simulink model "bio_matfunc_srp_torque_var"  (R2017b)
settings: Solver=VariableStepAuto  StartTime=0.0  StopTime=10.0  RelTol=1e-3
settings Model: Creator=ktrinh  LastModifiedBy=ktrinh

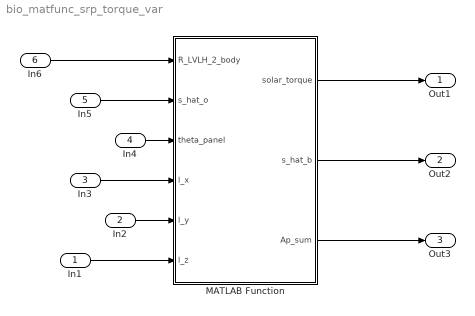
== system bio_matfunc_srp_torque_var ==
  In1 : Inport  OutDataTypeStr=double  PortDimensions=1
  In2 : Inport  Port=2  OutDataTypeStr=double  PortDimensions=1
  In3 : Inport  Port=3  OutDataTypeStr=double  PortDimensions=1
  In4 : Inport  Port=4  OutDataTypeStr=double  PortDimensions=1
  In5 : Inport  Port=5  OutDataTypeStr=double  PortDimensions=3
  In6 : Inport  Port=6  OutDataTypeStr=double  PortDimensions=[3,3]
  MATLAB Function : MATLAB Function  TreatAsAtomicUnit=on
  Out1 : Outport
  Out2 : Outport  Port=2
  Out3 : Outport  Port=3
  wires:
  In1/1 -> MATLAB Function/6(l_z)
  In2/1 -> MATLAB Function/5(l_y)
  In3/1 -> MATLAB Function/4(l_x)
  In4/1 -> MATLAB Function/3(theta_panel)
  In5/1 -> MATLAB Function/2(s_hat_o)
  MATLAB Function/1(solar_torque) -> Out1/1
  MATLAB Function/2(s_hat_b) -> Out2/1
  MATLAB Function/3(Ap_sum) -> Out3/1
  In6/1 -> MATLAB Function/1(R_LVLH_2_body)

== matlab function bio_matfunc_srp_torque_var/MATLAB Function ==
  data: R_LVLH_2_body input; solar_torque output; s_hat_o input; theta_panel input; l_x input; l_y input; l_z input; s_hat_b output; Ap_sum output
% function [solar_torque,s_hat_b] = srp_torque_var(R_LVLH_2_body,s_hat_o,theta_panel,l_x,l_y,l_z)
% %#codegen
% 
% Rob = R_LVLH_2_body;
% % this function calculates solar torque for a variable panel configuration
% % where the solar panels can rotate about the spacecraft y-axis
% % theta_panel is the angle in degrees that the panels are rotated from the
% % z axis -- i.e. theta_panel = 0 when panels are aligned normal to z axis
% 
% % Define constants
% SC = 1367;       % W/m^2, solar constant
% c = 3e8;         % m/s, speed of light
% q = 1;           % Reflectance
% 
% % Calculate an intermediate constant
% Fc = (SC/c)*(1+q);
% 
% % Define the surface areas associated with each face of the spacecraft.
% % Note that As_4 is the surface area for the 1U x 2U face of the spacecraft
% % with two 3U x 3U deployable arrays
% 
% %depending on position of panels, their contribution to surface area
% %changes
% %two boundaries: 1. nominal configuration where panels contribute full Ap
% %to z face
% %2. panels contribute full Ap to x face
% %between these two boundaries, panels contribute to both x and z surface
% %areas  with cosine relationship
% %area of two panels
% Apanel = 2*0.3*0.3;
% %Apanel = 0;
% 
% As_xp = l_y*l_z;
% As_xm = l_y*l_z;
% As_yp = l_x*l_z;
% As_ym = l_x*l_z;
% As_zp = l_x*l_y;
% As_zm = l_x*l_y;
% 
% As = [As_xp As_xm As_yp As_ym As_zp As_zm Apanel Apanel];
% 
% % Define the unit vector to the sun defined in the orbit frame
% s_hat_b = Rob*s_hat_o;
% 
% % Define a vector from the origin of the body frame to the center of
% % gravity of the spacecraft Cg
% 
% r_cg = 0.1*[-l_x; -l_y; -l_z];
% %r_cg = [0; 0; -l_z/3;];
% %r_cg = [0;0;0];
% 
% % Define vectors in the body frame describing the offset between Cp and Cg 
% % for each face of the spacecraft
% 
% r_cpxp = [l_x/2 0 0]';
% r_cpxm = [-l_x/2 0 0]';
% r_cpyp = [0 l_y/2 0]';
% r_cpym = [0 -l_y/2 0]';
% r_cpzp = [0 0 l_z/2]';
% r_cpzm = [0 0 -l_z/2]';
% 
% r_cp_panel = [0 0 l_z/2]';
% 
% r_cp = [r_cpxp r_cpxm r_cpyp r_cpym r_cpzp r_cpzm r_cp_panel r_cp_panel];
% 
% b_xp = [1 0 0]';
% b_xm = [-1 0 0]';
% b_yp = [0 1 0]';
% b_ym = [0 -1 0]';
% b_zp = [0 0 1]';
% b_zm = [0 0 -1]';
% 
% b_panel_p = [-sind(theta_panel) 0 cosd(theta_panel)]';
% b_panel_m = -1*b_panel_p;
% 
% b = [b_xp b_xm b_yp b_ym b_zp b_zm b_panel_p b_panel_m];
% 
% Ms_sum = [0 0 0]';
% for i = 1:8
%     dot_inc_ang = dot(s_hat_b,b(:,i))/norm(s_hat_b);
%     inc_ang = acos(dot_inc_ang);
% %     if isreal(dot_inc_ang) == 0
% %         inc_ang = 90*pi/180;
% %     else
% %         inc_ang = acos(dot_inc_ang);
% %     end
%     if inc_ang > 90*pi/180
%         inc_ang = 90*pi/180;
%     end
%     Ap = As(i)*cos(inc_ang);
%     Fs = Fc*Ap;
%     r_offset = r_cg - r_cp(:,i);
%     %r_offset = r_cp(:,i) - r_cg;
%     Ms = cross(r_offset,Fs*s_hat_b);
%     
%     Ms_sum = Ms_sum + Ms;
% end
% solar_torque = Ms_sum;










function [solar_torque,s_hat_b,Ap_sum] = srp_torque_var(R_LVLH_2_body,s_hat_o,theta_panel,l_x,l_y,l_z)
%#codegen

Rob = R_LVLH_2_body;
% this function calculates solar torque for a variable panel configuration
% where the solar panels can rotate about the spacecraft y-axis
% theta_panel is the angle in degrees that the panels are rotated from the
% z axis -- i.e. theta_panel = 0 when panels are aligned normal to z axis

% Define constants
SC = 1367;       % W/m^2, solar constant
c = 3e8;         % m/s, speed of light
q = 1;           % Reflectance

% Calculate an intermediate constant
Fc = (SC/c)*(1+q);

% Define the surface areas associated with each face of the spacecraft.
% Note that As_4 is the surface area for the 1U x 2U face of the spacecraft
% with two 3U x 3U deployable arrays

%depending on position of panels, their contribution to surface area
%changes
%two boundaries: 1. nominal configuration where panels contribute full Ap
%to z face
%2. panels contribute full Ap to x face
%between these two boundaries, panels contribute to both x and z surface
%areas  with cosine relationship
%area of two panels
Apanel = 0.3*0.3;
%Apanel = 0;

As_xp = l_y*l_z;
As_xm = l_y*l_z;
As_yp = l_x*l_z;
As_ym = l_x*l_z;
As_zp = l_x*l_y;
As_zm = l_x*l_y;

As = [As_xp As_xm As_yp As_ym As_zp As_zm Apanel Apanel Apanel Apanel];

% Define the unit vector to the sun defined in the orbit frame
s_hat_b = Rob*s_hat_o;

% Define a vector from the origin of the body frame to the center of
% gravity of the spacecraft Cg

r_cg = 0.1*[-l_x; -l_y; -l_z];
%r_cg = [0; 0; -l_z/3;];
%r_cg = [0;0;0];

% Define vectors in the body frame describing the offset between Cp and Cg 
% for each face of the spacecraft

r_cpxp = [l_x/2 0 0]';
r_cpxm = [-l_x/2 0 0]';
r_cpyp = [0 l_y/2 0]';
r_cpym = [0 -l_y/2 0]';
r_cpzp = [0 0 l_z/2]';
r_cpzm = [0 0 -l_z/2]';

r_cp_panel1_p = [0.25 0 l_z/2]';
r_cp_panel1_m = [0.25 0 l_z/2]';
r_cp_panel2_p = [-0.25 0 l_z/2]';
r_cp_panel2_m = [-0.25 0 l_z/2]';

r_cp = [r_cpxp r_cpxm r_cpyp r_cpym r_cpzp r_cpzm r_cp_panel1_p r_cp_panel1_m r_cp_panel2_p r_cp_panel2_m];

b_xp = [1 0 0]';
b_xm = [-1 0 0]';
b_yp = [0 1 0]';
b_ym = [0 -1 0]';
b_zp = [0 0 1]';
b_zm = [0 0 -1]';

b_panel_p = [-sind(theta_panel) 0 cosd(theta_panel)]';
b_panel_m = -1*b_panel_p;

b = [b_xp b_xm b_yp b_ym b_zp b_zm b_panel_p b_panel_m b_panel_p b_panel_m];

Ms_sum = [0 0 0]';
Ap_sum = zeros(10,1);
for i = 1:10
    dot_inc_ang = dot(s_hat_b,b(:,i))/norm(s_hat_b);
    inc_ang = acos(dot_inc_ang);
%     if isreal(dot_inc_ang) == 0
%         inc_ang = 90*pi/180;
%     else
%         inc_ang = acos(dot_inc_ang);
%     end
    if inc_ang > 90*pi/180
        inc_ang = 90*pi/180;
    end
        
    Ap = As(i)*cos(inc_ang);
    
    Ap_sum(i) = Ap;
    
    Fs = Fc*Ap;
    r_offset = r_cg - r_cp(:,i);
    %r_offset = r_cp(:,i) - r_cg;
    Ms = cross(r_offset,Fs*s_hat_b);
    
    Ms_sum = Ms_sum + Ms;
end
solar_torque = Ms_sum;
